simulink model "MODELBLDC2020"  (R2019b)
settings: Solver=VariableStepAuto  StartTime=0.0  StopTime=0.75  RelTol=1e-3
libraries: powerlib x6, fuzblock x1, eePwmGenerator x1
settings Model: Creator=Toan Thanh Nguyen  LastModifiedBy=ayush
settings SolverCC: ZeroCrossAlgorithm=Adaptive
settings DebuggingCC: IgnoredZcDiagnostic=none
settings SFSimCC: CustomCodeUndefinedFunction=UseInterfaceOnly

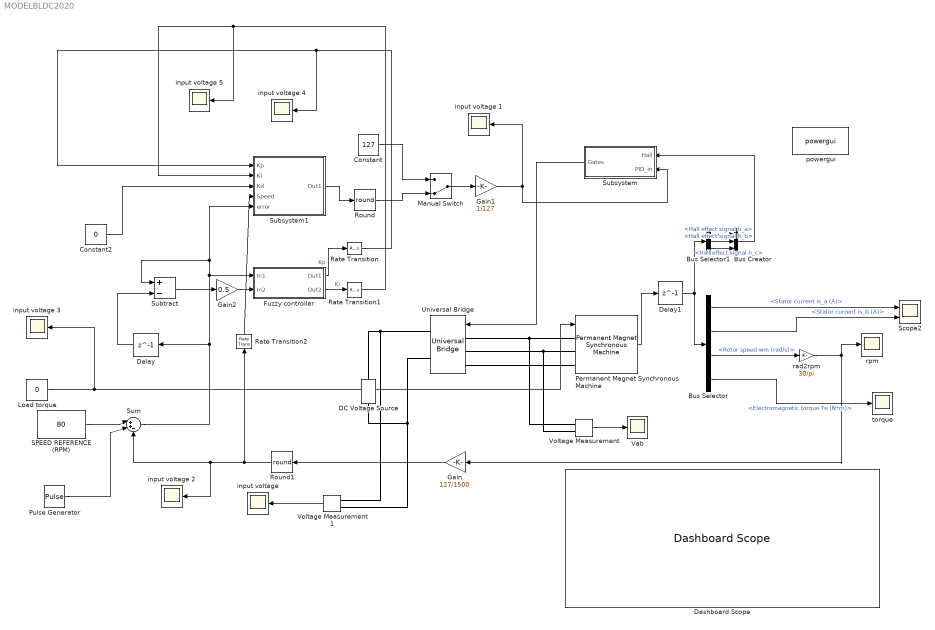
== system MODELBLDC2020 ==
  Bus Creator : BusCreator  Inputs=3
  Bus Selector : BusSelector  OutputSignals=Stator current is_a (A),Stator current is_b (A),Rotor speed wm (rad/s),Electromagnetic torque Te (N*m)
  Bus Selector1 : BusSelector  OutputSignals=Hall effect signal h_a,Hall effect signal h_b,Hall effect signal h_c
  Constant : Constant  Value=127
  Constant2 : Constant  Value=0
  DC Voltage Source : powerlib/Electrical Sources/DC Voltage Source  Amplitude=12  Measurements=None
      settings: SourceProductName=Simscape Electrical
  Dashboard Scope : DashboardScope
  Delay : Delay  DelayLength=1
  Delay1 : Delay  DelayLength=1
  Fuzzy controller : Subsystem
  Gain : Gain  Gain=127/1500
  Gain1 : Gain  Gain=1/127
  Gain2 : Gain  Gain=0.5
  "Load torque " : Constant  Value=0
  Manual Switch : ManualSwitch  CurrentSetting=0
  Permanent Magnet Synchronous Machine : powerlib/Machines/Permanent Magnet Synchronous Machine  NbPhases=3  FluxDistribution=Trapezoidal  RotorType=Round  MechanicalLoad=Torque Tm  PresetModel=No  ShowDetailedParameters=on  MeasurementBus=off  Resistance=0.515  Inductance=0.000286  dqInductances=[8.5e-3,8.5e-3]  La=0.000395  MachineConstant=Flux linkage established by magnets (V.s)  Flux=0.00209375  VoltageCst=3.5081  TorqueCst=0.0335  Flat=120  Mechanical=[1.35e-05 0.00108862 8]  PolePairs=4  InitialConditions=[0,0, 0,0]  InitialConditions5ph=[0 0 0 0 0 0]  RefAngle=90 degrees behind phase A axis (modified Park)  IterativeDiscreteModel=Trapezoidal non iterative  TsBlock=-1  TsPowergui=0
  Pulse Generator : DiscretePulseGenerator  PulseType=Time based  Amplitude=-40  Period=10  PulseWidth=50  PhaseDelay=0.15
  Rate Transition : RateTransition
  Rate Transition1 : RateTransition
  Rate Transition2 : RateTransition
  Round : Rounding  Operator=round
  Round1 : Rounding  Operator=round
  "SPEED REFERENCE (RPM) " : Constant  Value=80
  Scope2 : Scope  NumInputPorts=2
  Subsystem : Subsystem
  Subsystem1 : Subsystem
  Subtract : Sum  Inputs=+-
  Sum : Sum  Inputs=|++-
  Universal Bridge : powerlib/Power Electronics/Universal Bridge  Arms=3  SnubberResistance=1e5  SnubberCapacitance=inf  Device=MOSFET / Diodes  Ron=1e-3  Lon=0  ForwardVoltages="[  0  0  ]"  ForwardVoltage=0  GTOparameters=[ 10e-6 , 20e-6 ]  IGBTparameters=[ 1e-6 , 2e-6 ]  Measurements=None  Measurements_2=None  converterType=Rectifier
      settings: SourceProductName=Simscape Electrical
  Vab : Scope
  Voltage Measurement : powerlib/Measurements/Voltage Measurement  PhasorSimulation=off  OutputType=Complex  PSBequivalent=0
      settings: SourceProductName=Simscape Electrical
  Voltage Measurement1 : powerlib/Measurements/Voltage Measurement  PhasorSimulation=off  OutputType=Complex  PSBequivalent=0
      settings: SourceProductName=Simscape Electrical
  input voltage {,1..5} (6 alike) : Scope
  powergui : powerlib/powergui  Priority=1  SimulationMode=Discrete  SampleTime=1e-5  frequency=60  Iterations=50  frequencyindice=0  Pbase=100e6  ErrMax=1e-4  UnitsV=kV  UnitsW=MW  buscounter=0  FunctionMessages=off  echomessages=off  EnableUseOfTLC=off  CurrentSourceSwitches=off  DisableSnubberDevices=off  DisableRonSwitches=off  DisableVfSwitches=off  DisplayEquations=off  AutomaticDiscreteSolvers=off  SolverType=Tustin/Backward Euler (TBE)  Interpol=off  ExternalGateDelay=off  methode=off  Ts=100  x0status=blocks  SPID=on  SwTol=0  HookPort=off  NonlinearTolerance=0  nMaxIteration=15  ContinueOnMaxIteration=off  RestoreLinks=warning  ResistiveCurrentMeasurement=off  Frange=[0:2:500]  Ylog=off  Xlog=on  ShowGrid=off  save=off  variable=ZData  structure=0  ZoomFFT=off  StartTime=0.0  cycles=1  DisplayStyle=1  fundamental=60  FreqAxis=off  MaxFrequency=1000  frequencyindicesteady=1  RmsSteady=1  display=off
      settings: SourceProductName=Simscape Electrical
  rad2rpm : Gain  Gain=30/pi
  "rpm " : Scope
  torque : Scope
  wires:
  Sum/1 -> Subtract/1, Subsystem1/5(error), Fuzzy controller/1(In1), Delay/1
  "SPEED REFERENCE (RPM) "/1 -> Sum/1
  Subsystem/1(Gates) -> Universal Bridge/1
  "Load torque "/1 -> input voltage 3/1, Permanent Magnet Synchronous Machine/1
  Bus Selector/1 -> Scope2/1  "<Stator current is_a (A)>"
  Bus Selector/2 -> Scope2/2  "<Stator current is_b (A)>"
  Bus Selector/3 -> rad2rpm/1  "<Rotor speed wm (rad/s)>"
  Bus Selector/4 -> torque/1  "<Electromagnetic torque Te (N*m)>"
  rad2rpm/1 -> "rpm "/1, Gain/1
  Voltage Measurement/1 -> Vab/1
  Bus Selector1/1 -> Bus Creator/1  "<Hall effect signal h_a>"
  Bus Selector1/2 -> Bus Creator/2  "<Hall effect signal h_b>"
  Bus Selector1/3 -> Bus Creator/3  "<Hall effect signal h_c>"
  Bus Creator/1 -> Subsystem/1(Hall)
  Voltage Measurement1/1 -> "input voltage "/1
  Constant/1 -> Manual Switch/1
  Manual Switch/1 -> Gain1/1
  Gain/1 -> Round1/1
  Gain1/1 -> input voltage 1/1, Subsystem/2(PID_in)
  Round/1 -> Manual Switch/2
  Gain2/1 -> Fuzzy controller/2(In2)
  Subtract/1 -> Gain2/1
  Delay/1 -> Subtract/2
  Fuzzy controller/1(Out1) -> Rate Transition/1  "Kp"
  Subsystem1/1(Out1) -> Round/1
  Constant2/1 -> Subsystem1/3(Kd)
  Permanent Magnet Synchronous Machine/1 -> Delay1/1
  Pulse Generator/1 -> Sum/2
  Round1/1 -> Rate Transition2/1, Sum/3, input voltage 2/1
  Fuzzy controller/2(Out2) -> Rate Transition1/1  "Ki"
  Delay1/1 -> Bus Selector1/1, Bus Selector/1
  Rate Transition2/1 -> Subsystem1/4(Speed)
  Rate Transition/1 -> Subsystem1/1(Kp), input voltage 4/1
  Rate Transition1/1 -> Subsystem1/2(KI), input voltage 5/1
  connections:
  Universal Bridge/LConn2 -- Voltage Measurement/LConn2 -- Permanent Magnet Synchronous Machine/LConn2
  Universal Bridge/LConn1 -- Voltage Measurement/LConn1 -- Permanent Magnet Synchronous Machine/LConn1
  Universal Bridge/LConn3 -- Permanent Magnet Synchronous Machine/LConn3
  Voltage Measurement1/LConn1 -- DC Voltage Source/RConn1 -- Universal Bridge/RConn1
  Voltage Measurement1/LConn2 -- DC Voltage Source/LConn1 -- Universal Bridge/RConn2

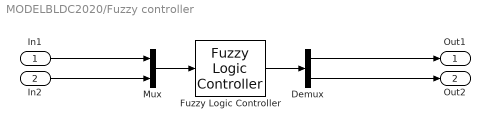
== system MODELBLDC2020/Fuzzy controller ==
  In1 : Inport
  In2 : Inport  Port=2
  Demux : Demux  Outputs=2
  Fuzzy Logic Controller : fuzblock/Fuzzy Logic  Controller  FIS='fuzzytest.fis'  OutputSampleNumber=101  DataType=double  FuzzifiedInputs=off  RuleFiringStrengths=off  RuleOutputs=off  AggregatedOutputs=off  SimulateUsing=Interpreted execution  OutOfRangeInputValueMessage=warning  NoRuleFiredMessage=warning  EmptyOutputFuzzySetMessage=warning
  Mux : Mux  Inputs=2
  Out1 : Outport
  Out2 : Outport  Port=2
  wires:
  Mux/1 -> Fuzzy Logic Controller/1
  Fuzzy Logic Controller/1 -> Demux/1
  In1/1 -> Mux/1
  In2/1 -> Mux/2
  Demux/1 -> Out1/1
  Demux/2 -> Out2/1

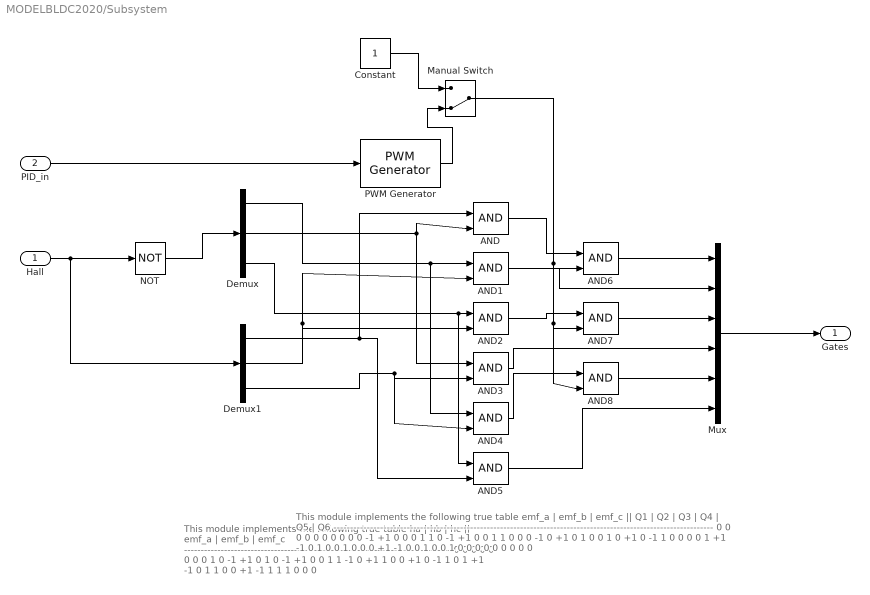
== system MODELBLDC2020/Subsystem ==
  note: This module implements the following true table
      |
      |    ha   |   hb   |   hc   ||   emf_a   |   emf_b   |   emf_c
      |     --------------------------------------------------------------------------------
      | 0          0         0          0               0               0
      | 0          0         1          0               -1              +1
      | 0          1         0          -1              +1                0
      | 0          1         1          -1               0               +1
      | 1          0         0         +1               0               -1
      | 1          0         1         +1              -1                0
      | 1          1         0          0              +1               -1
      | 1          1         1          0               0                0
  note: This module implements the following true table
      |
      |    emf_a   |   emf_b   |   emf_c   ||   Q1   |   Q2   |   Q3   |   Q4   |   Q5   |   Q6
      |     ------------------------------------------------------------------------------------------------------------------
      |       0              0                0            0          0          0           0        0        0
      |       0               -1              +1          0          0          0           1        1        0
      |     -1              +1                0          0          1          1           0        0        0
      |     -1               0               +1          0          1         0           0        1        0
      |    +1               0                -1          1          0          0           0        0        1
      |    +1              -1                0           1          0          0           1        0        0
      |      0              +1               -1           0          0          1           0        0        1
      |     0              0                0             0          0          0           0        0        0
  Hall : Inport
  PID_in : Inport  Port=2
  AND{,1..8} (9 alike) : Logic  IconShape=distinctive  AllPortsSameDT=off  OutDataTypeStr=boolean
  Constant : Constant
  Demux : Demux  Outputs=3
  Demux1 : Demux  Outputs=3
  Manual Switch : ManualSwitch  CurrentSetting=0
  Mux : Mux  Inputs=6
  NOT : Logic  Operator=NOT  IconShape=distinctive  AllPortsSameDT=off  OutDataTypeStr=boolean
  PWM Generator : eePwmGenerator/PWM Generator  CarrCount=Up  Tper=1e-4  Ts=1e-6
      settings: SourceProductName=Simscape Electrical
  Gates : Outport
  wires:
  NOT/1 -> Demux/1
  Hall/1 -> Demux1/1, NOT/1
  Mux/1 -> Gates/1
  AND1/1 -> Mux/2
  AND3/1 -> Mux/4
  AND5/1 -> Mux/6
  Demux1/1 -> AND5/2, AND/1
  Demux/2 -> AND3/1, AND/2
  Demux/1 -> AND4/1, AND1/1
  Demux1/2 -> AND2/2, AND1/2
  Demux/3 -> AND5/1, AND2/1
  Demux1/3 -> AND4/2, AND3/2
  AND7/1 -> Mux/3
  AND2/1 -> AND7/1
  AND6/1 -> Mux/1
  AND/1 -> AND6/1
  AND8/1 -> Mux/5
  AND4/1 -> AND8/1
  PWM Generator/1 -> Manual Switch/2
  PID_in/1 -> PWM Generator/1
  Constant/1 -> Manual Switch/1
  Manual Switch/1 -> AND6/2, AND8/2, AND7/2

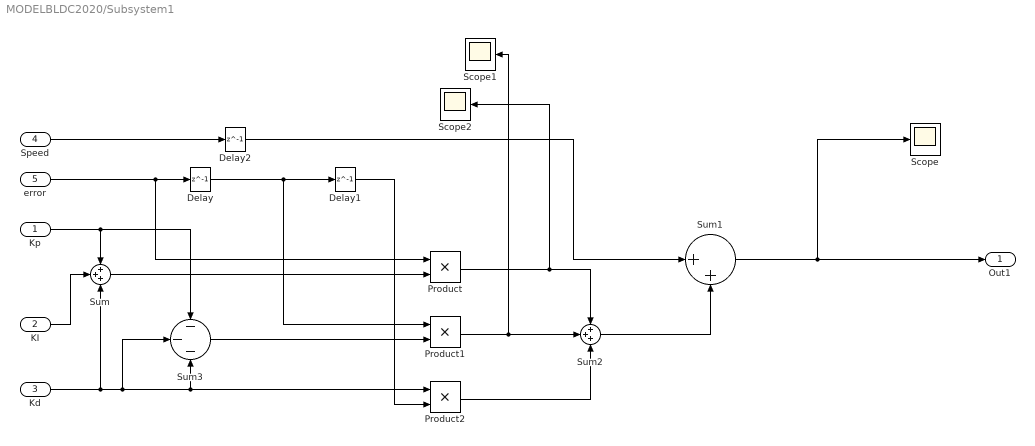
== system MODELBLDC2020/Subsystem1 ==
  Kp : Inport
  KI : Inport  Port=2
  Kd : Inport  Port=3
  Speed : Inport  Port=4
  error : Inport  Port=5
  Delay : Delay  DelayLength=1
  Delay1 : Delay  DelayLength=1
  Delay2 : Delay  DelayLength=1
  Product : Product
  Product1 : Product
  Product2 : Product
  Scope : Scope
  Scope1 : Scope
  Scope2 : Scope
  Sum : Sum  Inputs=+++
  Sum1 : Sum  Inputs=|++
  Sum2 : Sum  Inputs=+++
  Sum3 : Sum  Inputs=---
  Out1 : Outport
  wires:
  error/1 -> Product/1, Delay/1
  Delay/1 -> Product1/1, Delay1/1
  Sum/1 -> Product/2
  Kp/1 -> Sum3/1, Sum/1
  KI/1 -> Sum/2
  Kd/1 -> Sum3/2, Sum3/3, Product2/1, Sum/3
  Delay1/1 -> Product2/2
  Sum1/1 -> Scope/1, Out1/1
  Product1/1 -> Scope1/1, Sum2/2
  Product/1 -> Scope2/1, Sum2/1
  Product2/1 -> Sum2/3
  Sum2/1 -> Sum1/2
  Sum3/1 -> Product1/2
  Speed/1 -> Delay2/1
  Delay2/1 -> Sum1/1
